simulink model "IPModelNonlinearSystemHomoclinicOrbit"  (R2024a)
settings: Solver=FixedStepAuto  StartTime=0.0  StopTime=80  FixedStep=.01  RelTol=1e-3
PreLoadFcn:
  | m  = .164948;
  | M = 1.035052;
  | l = 0.2425;
  | kdx = 1;
  | kv = 1;
  | kE = 1;
  | kx = 1/100;
  | g = 9.804;
  | 
  | % kdx = kdx*10;
  | % kv = kv*10;
  | % kE = kE*10;
  | % kx = kx*10;
  | %
  | % kdx = kdx*1000;
  | % kv = kv*1000;
  | % kE = kE*1000;
  | % kx = kx*1000;
  | 
  | x0 = 0;
  | dx0 = 0;
  | theta0 = 23*D2R;
  | dtheta0 = 0;
  | 
  | ml = m*l;
  | ml2 = ml*l;
  | 
  | 
  | phi = 25; %error from upright pos, in degrees
  | R2D = 180/pi;
  | D2R = pi/180;
  | 
  | 
  | A = 1/(M*l)*[0 , 1, 0, 0;
  |           0, 0, -m*l*g, 0;
  |           0, 0, 0, 1;
  |           0, 0, (M+m)*g, 0];
  | B = 1/(M*l)*[0;
  |             l;
  |             0;
  |             -1];
  | 
  | C = [1,0,0,0;
  |     0,0,1,0];
  | 
  | D = [0;0];
values from neighbouring files (symbols this model uses):
  K = lqr(A,B,Q,R)    [IPdynamicsHomoclinicOrbitStabilization.m]    (also in invertedPendulumDynamics.m = [-31.6228, -22.4894, 87.1251, 18.1589])
libraries: vrlib x3, simulink x1
settings Model: NumberOfSteps=2  SnapshotBufferSize=5  SnapshotInterval=5  Creator=rahelmizrahi  LastModifiedBy=rahelmizrahi
settings SolverCC: ZeroCrossAlgorithm=Adaptive
settings DebuggingCC: IgnoredZcDiagnostic=none

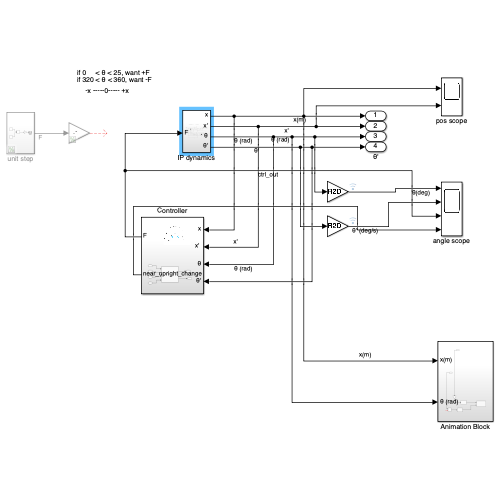
[thumbnail: Simulink's stored preview of the top-level diagram]
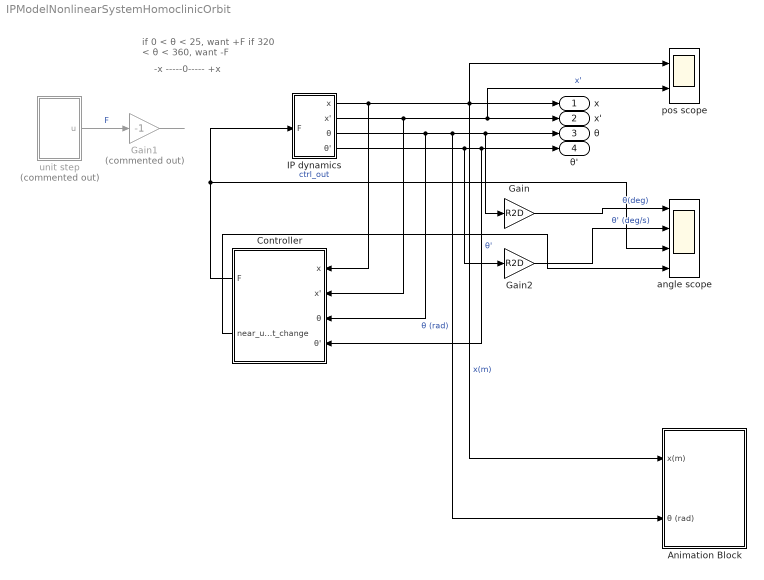
== system IPModelNonlinearSystemHomoclinicOrbit ==
  note: if 0     < θ < 25, want +F
      | if 320 < θ < 360, want -F
  note: -x -----0----- +x
  Animation Block : Subsystem
  Controller : Subsystem
  Gain : Gain  Gain=R2D
  Gain1 : Gain  Commented=on  Gain=-1
  Gain2 : Gain  Gain=R2D
  IP dynamics : Subsystem
  angle scope : Scope  NumInputPorts=4
  pos scope : Scope  NumInputPorts=2
  unit step : Subsystem  Commented=on
  x : Outport
  x' : Outport  Port=2
  θ : Outport  Port=3
  θ' : Outport  Port=4
  wires:
  Gain1/1 -> ?
  IP dynamics/2(x') -> Controller/2("x' "), pos scope/2, x'/1  "x'"
  IP dynamics/4(θ') -> Gain2/1, Controller/4(θ'), θ'/1  "θ'"
  unit step/1(u) -> Gain1/1  "F"
  Gain2/1 -> angle scope/2  "θ' (deg/s)"
  Gain/1 -> angle scope/1  "θ(deg)"
  IP dynamics/3(θ) -> Controller/3(θ), Gain/1, θ/1, Animation Block/2(θ (rad))  "θ (rad)"
  IP dynamics/1(x) -> Animation Block/1(x(m)), pos scope/1, x/1, Controller/1(x)  "x(m)"
  Controller/1(F) -> angle scope/3, IP dynamics/1(F)  "ctrl_out"
  Controller/2(near_upright_change) -> angle scope/4

== system IPModelNonlinearSystemHomoclinicOrbit/Animation Block ==
  x(m) : Inport
  θ (rad) : Inport  Port=2
  Add : Sum
  Gain6 : Gain  Gain=10
  VR Sink1 : vrlib/VR Sink  InstantiateOnLoad=on  SampleTime=0.1  ViewEnable=on  RemoteChange=off  RemoteView=off  FieldsWritten=cart.translation.3.1.1.double#joint.rotation.4.1.1.double  WorldFileName=/Users/rahelmizrahi/Downloads/upload 2/Inverted_pendulum12.wrl  AutoView=on  VideoDimensions=[]  AllowVariableSize=off  FigureProperties="{'Position', 'Name', 'Viewpoint', 'CameraBound', 'CameraDirection', 'CameraPosition', 'CameraUpVector', 'ZoomFactor', 'Antialiasing', 'Headlight', 'Lighting', 'Sound', 'StatusBar', 'Stereo3D', 'Stereo3DCameraOffset', 'Stereo3DHIT', 'ToolBar', 'Textures', 'Transparency', 'Triad', 'Wireframe', 'NavZones', 'NavMode', 'NavSpeed', 'CaptureFileFormat', 'CaptureFileName', 'Record2DCompressMethod', 'Record2DCompressQuality', 'Record2D', 'Record2DFileName', 'Record2DFPS', 'NavPanel'; [5.0000000000000000e+00   1.0300000000000000e+02   5.7600000000000000e+02   3.5000000000000000e+02], '', '', 'on', [0.0000000000000000e+00   0.0000000000000000e+00  -9.9999999999999989e-01], [0.0000000000000000e+00  -6.0000002384185791e-01   2.6254408740997309e+01], [0.0000000000000000e+00   1.0000000000000000e+00   0.0000000000000000e+00], [1.0000000000000000e+00], 'on', 'on', 'on', 'on', 'on', 'off', [1.0000000149011612e-01], [0.0000000000000000e+00], 'on', 'on', 'on', 'none', 'off', 'off', 'fly', 'normal', 'tif', '%f_anim_%n.tif', 'auto', [7.5000000000000000e+01], 'off', '%f_anim_%n.avi', 'auto', 'halfbar'}"
  angle sig expander : vrlib/VR Signal Expander  outwidth=4  outidx=4
  pos sig expander : vrlib/VR Signal Expander  outwidth=3  outidx=1
  wires:
  θ (rad)/1 -> Add/1
  pos sig expander/1 -> VR Sink1/1
  Add/1 -> angle sig expander/1
  ? -> Add/2
  Gain6/1 -> pos sig expander/1
  angle sig expander/1 -> VR Sink1/2
  x(m)/1 -> Gain6/1

== system IPModelNonlinearSystemHomoclinicOrbit/Controller ==
  x : Inport
  "x' " : Inport  Port=2
  θ : Inport  Port=3
  θ' : Inport  Port=4
  ctrl switch : Subsystem
  F : Outport
  near_upright_change : Outport  Port=2
  wires:
  ctrl switch/1(control_out) -> F/1  "F"
  "x' "/1 -> ctrl switch/4("x' ")  "x'"
  x/1 -> ctrl switch/3(x)  "x"
  θ'/1 -> ctrl switch/2(θ')  "θ'"
  θ/1 -> ctrl switch/1(θ)  "θ"
  ctrl switch/2(near_upright_change) -> near_upright_change/1

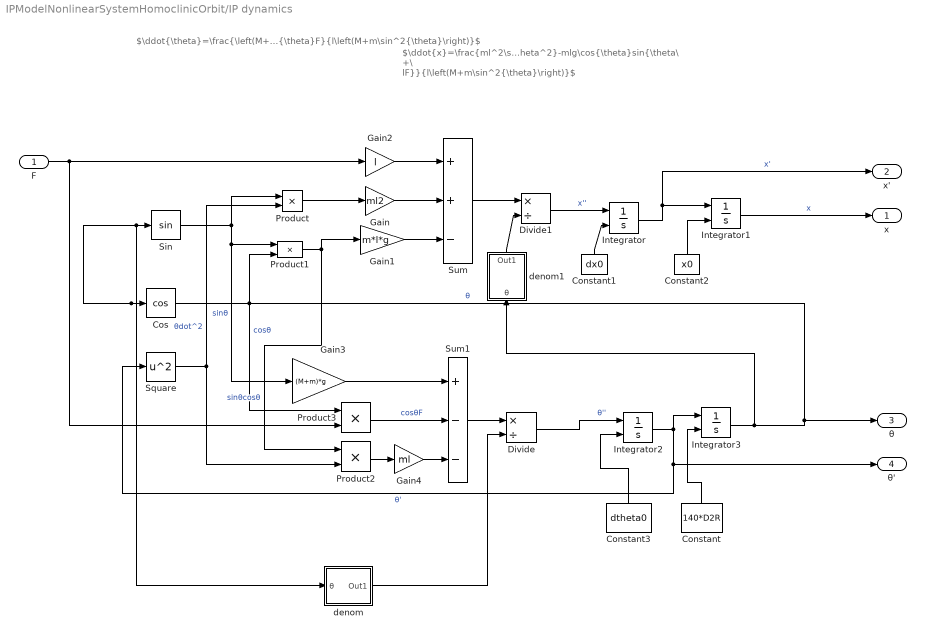
== system IPModelNonlinearSystemHomoclinicOrbit/IP dynamics ==
  note: $\ddot{\theta}=\frac{\left(M+m\right)g\sin{\theta-ml\sin{\theta}\cos{\theta}\dot{\theta^2}}-\cos{\theta}F}{l\left(M+m\sin^2{\theta}\right)}$
  note: $\ddot{x}=\frac{ml^2\sin{\theta}\dot{\theta^2}-mlg\cos{\theta}sin{\theta\ +\ lF}}{l\left(M+m\sin^2{\theta}\right)}$
  F : Inport
  Constant : Constant  Value=140*D2R
  Constant1 : Constant  Value=dx0
  Constant2 : Constant  Value=x0
  Constant3 : Constant  Value=dtheta0
  Cos : Trigonometry  Operator=cos
  Divide : Product  Inputs=*/
  Divide1 : Product  Inputs=*/
  Gain : Gain  Gain=ml2
  Gain1 : Gain  Gain=m*l*g
  Gain2 : Gain  Gain=l
  Gain3 : Gain  Gain=(M+m)*g
  Gain4 : Gain  Gain=ml
  Integrator : Integrator  InitialConditionSource=external
  Integrator1 : Integrator  InitialConditionSource=external
  Integrator2 : Integrator  InitialConditionSource=external
  Integrator3 : Integrator  InitialConditionSource=external  WrappedStateUpperValue=2*pi  WrappedStateLowerValue=0
  Product{,1..3} (4 alike) : Product
  Sin : Trigonometry
  Square : Math  Operator=square
  Sum : Sum  Inputs=++-
  Sum1 : Sum  Inputs=+--
  denom : Subsystem
  denom1 : Subsystem
  x : Outport
  x' : Outport  Port=2
  θ : Outport  Port=3
  θ' : Outport  Port=4
  wires:
  Product/1 -> Gain/1
  Sum1/1 -> Divide/1
  F/1 -> Product3/2, Gain2/1
  Gain2/1 -> Sum/1
  Product1/1 -> Product2/1, Gain1/1  "sinθcosθ"
  Product3/1 -> Sum1/2  "cosθF"
  Gain1/1 -> Sum/3
  Integrator1/1 -> x/1  "x"
  Square/1 -> Product/2, Product2/2  "θdot^2"
  Cos/1 -> Product1/2, Product3/1  "cosθ"
  Integrator2/1 -> Integrator3/1, θ'/1, Square/1  "θ'"
  Integrator3/1 -> denom1/1(θ), θ/1, denom/1(θ), Sin/1, Cos/1  "θ"
  Gain3/1 -> Sum1/1
  Gain/1 -> Sum/2
  Product2/1 -> Gain4/1
  Sin/1 -> Gain3/1, Product1/1, Product/1  "sinθ"
  Integrator/1 -> x'/1, Integrator1/1  "x'"
  Sum/1 -> Divide1/1
  Gain4/1 -> Sum1/3
  Constant/1 -> Integrator3/2
  Constant1/1 -> Integrator/2
  Constant2/1 -> Integrator1/2
  Constant3/1 -> Integrator2/2
  Divide/1 -> Integrator2/1  "θ''"
  denom/1(Out1) -> Divide/2
  Divide1/1 -> Integrator/1  "x''"
  denom1/1(Out1) -> Divide1/2

== system IPModelNonlinearSystemHomoclinicOrbit/unit step ==
  Add : Sum  Inputs=-+
  Gain : Gain  Gain=10
  Step : Step  SampleTime=0
  Step1 : Step  Time=1.1  SampleTime=0
  u : Outport
  wires:
  Step1/1 -> Add/1
  Gain/1 -> u/1
  Step/1 -> Add/2
  Add/1 -> Gain/1

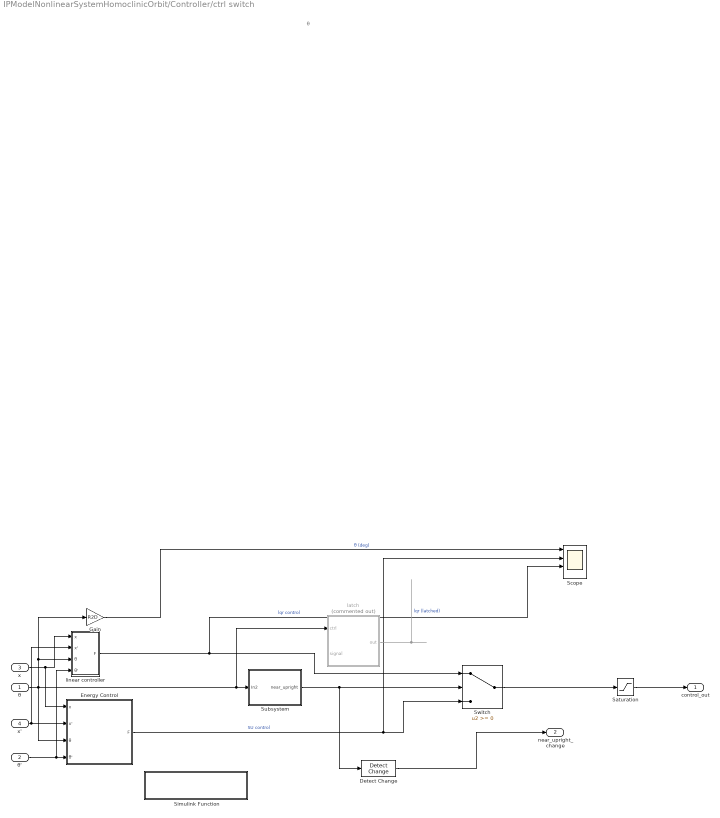
== system IPModelNonlinearSystemHomoclinicOrbit/Controller/ctrl switch ==
  note: θ
  θ : Inport
  θ' : Inport  Port=2
  x : Inport  Port=3
  "x' " : Inport  Port=4
  Detect Change : simulink/Logic and Bit Operations/Detect Change  vinit=0  OutDataTypeStr=boolean
  Energy Control : Subsystem
  Gain : Gain  Gain=R2D
  Saturation : Saturate  UpperLimit=6  LowerLimit=-6
  Scope : Scope  NumInputPorts=4
  Simulink Function : Subsystem  TreatAsAtomicUnit=on
  Subsystem : Subsystem
  Switch : Switch  SaturateOnIntegerOverflow=off  InputSameDT=off
  latch : Subsystem  Commented=on
  linear controller : Subsystem
  control_out : Outport
  near_upright_change : Outport  Port=2
  wires:
  Subsystem/1(near_upright) -> Detect Change/1, Switch/2
  Energy Control/1(F) -> Scope/2, Switch/3  "SU control"
  θ'/1 -> linear controller/4(θ'), Energy Control/4(θ')
  linear controller/1(F) -> Scope/3, Switch/1  "lqr control"
  "x' "/1 -> linear controller/2(x'), Energy Control/2(x')
  x/1 -> linear controller/1(x), Energy Control/1(x)
  θ/1 -> linear controller/3(θ), Gain/1, Energy Control/3(θ), latch/1(ctrl), Subsystem/1(In2)
  latch/1(out) -> ?  "lqr (latched)"
  Gain/1 -> Scope/1  "θ (deg)"
  Detect Change/1 -> near_upright_change/1
  Switch/1 -> Saturation/1
  Saturation/1 -> control_out/1

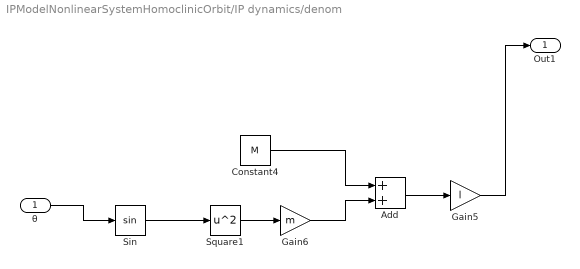
== system IPModelNonlinearSystemHomoclinicOrbit/IP dynamics/denom ==
  θ : Inport
  Add : Sum
  Constant4 : Constant  Value=M
  Gain5 : Gain  Gain=l
  Gain6 : Gain  Gain=m
  Sin : Trigonometry
  Square1 : Math  Operator=square
  Out1 : Outport
  wires:
  Gain5/1 -> Out1/1
  Square1/1 -> Gain6/1
  θ/1 -> Sin/1
  Constant4/1 -> Add/1
  Add/1 -> Gain5/1
  Gain6/1 -> Add/2
  Sin/1 -> Square1/1

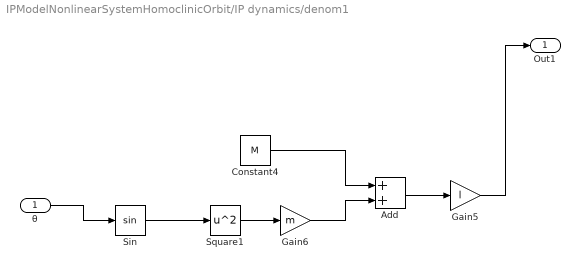
== system IPModelNonlinearSystemHomoclinicOrbit/IP dynamics/denom1 ==
  θ : Inport
  Add : Sum
  Constant4 : Constant  Value=M
  Gain5 : Gain  Gain=l
  Gain6 : Gain  Gain=m
  Sin : Trigonometry
  Square1 : Math  Operator=square
  Out1 : Outport
  wires:
  Gain5/1 -> Out1/1
  Square1/1 -> Gain6/1
  θ/1 -> Sin/1
  Constant4/1 -> Add/1
  Add/1 -> Gain5/1
  Gain6/1 -> Add/2
  Sin/1 -> Square1/1

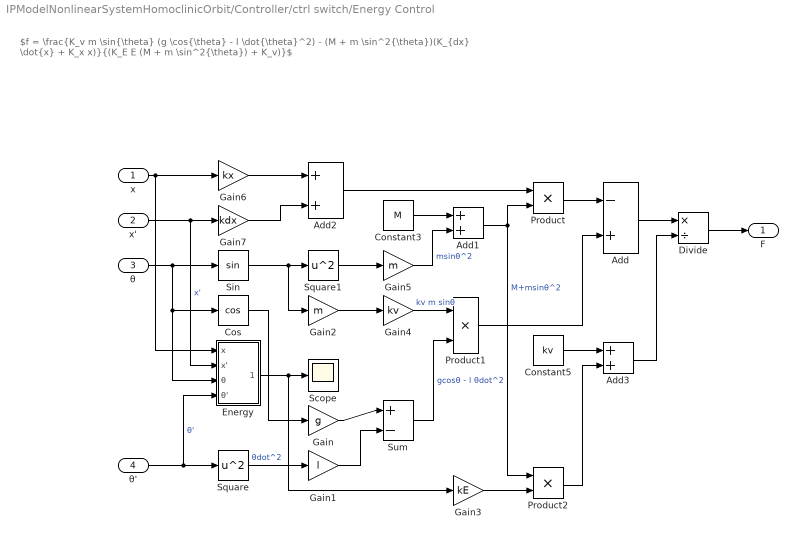
== system IPModelNonlinearSystemHomoclinicOrbit/Controller/ctrl switch/Energy Control ==
  note: $f = \frac{K_v m \sin{\theta} (g \cos{\theta} - l \dot{\theta}^2) - (M + m \sin^2{\theta})(K_{dx} \dot{x} + K_x x)}{(K_E E (M + m \sin^2{\theta}) + K_v)}$
  x : Inport
  x' : Inport  Port=2
  θ : Inport  Port=3
  θ' : Inport  Port=4
  Add : Sum  Inputs=-+
  Add1 : Sum
  Add2 : Sum
  Add3 : Sum
  Constant3 : Constant  Value=M
  Constant5 : Constant  Value=kv
  Cos : Trigonometry  Operator=cos
  Divide : Product  Inputs=*/
  Energy : Subsystem
  Gain : Gain  Gain=g
  Gain1 : Gain  Gain=l
  Gain2 : Gain  Gain=m
  Gain3 : Gain  Gain=kE
  Gain4 : Gain  Gain=kv
  Gain5 : Gain  Gain=m
  Gain6 : Gain  Gain=kx
  Gain7 : Gain  Gain=kdx
  Product : Product
  Product1 : Product
  Product2 : Product
  Scope : Scope
  Sin : Trigonometry
  Square : Math  Operator=square
  Square1 : Math  Operator=square
  Sum : Sum  Inputs=|+-
  F : Outport
  wires:
  Add/1 -> Divide/1
  Gain3/1 -> Product2/2
  Square/1 -> Gain1/1  "θdot^2"
  Add1/1 -> Product/2, Product2/1  "M+msinθ^2"
  Product/1 -> Add/1
  Sum/1 -> Product1/2  "gcosθ - l θdot^2"
  Gain4/1 -> Product1/1  "kv m sinθ"
  θ/1 -> Energy/3(θ), Cos/1, Sin/1
  Constant3/1 -> Add1/1
  Gain1/1 -> Sum/2
  Gain/1 -> Sum/1
  Add3/1 -> Divide/2
  x'/1 -> Energy/2(x'), Gain7/1  "x'"
  Product1/1 -> Add/2
  Gain2/1 -> Gain4/1
  Cos/1 -> Gain/1
  Add2/1 -> Product/1
  Gain6/1 -> Add2/1
  Square1/1 -> Gain5/1
  Energy/1(Energy) -> Scope/1, Gain3/1
  Gain7/1 -> Add2/2
  Product2/1 -> Add3/2
  Constant5/1 -> Add3/1
  θ'/1 -> Square/1, Energy/4(θ')  "θ'"
  Gain5/1 -> Add1/2  "msinθ^2"
  Divide/1 -> F/1
  x/1 -> Energy/1(x), Gain6/1
  Sin/1 -> Gain2/1, Square1/1

== system IPModelNonlinearSystemHomoclinicOrbit/Controller/ctrl switch/Simulink Function ==
  between : TriggerPort  TriggerType=function-call  IsSimulinkFunction=on  FunctionName=between  FunctionVisibility=scoped  VariantControl=(inherit)
  AND : Logic  IconShape=distinctive  AllPortsSameDT=off  OutDataTypeStr=boolean
  Relational Operator : RelationalOperator  OutDataTypeStr=boolean  RndMeth=Simplest  InputSameDT=off
  Relational Operator1 : RelationalOperator  Operator=<=  OutDataTypeStr=boolean  RndMeth=Simplest  InputSameDT=off
  input : ArgIn  DisableCoverage=on  ArgumentName=input
  min : ArgIn  Port=2  ArgumentName=min
  max : ArgIn  Port=3  ArgumentName=max
  out : ArgOut  DisableCoverage=on  OutDataTypeStr=boolean  ArgumentName=out
  wires:
  input/1 -> Relational Operator1/1, Relational Operator/1
  Relational Operator/1 -> AND/1
  Relational Operator1/1 -> AND/2
  AND/1 -> out/1
  min/1 -> Relational Operator/2
  max/1 -> Relational Operator1/2

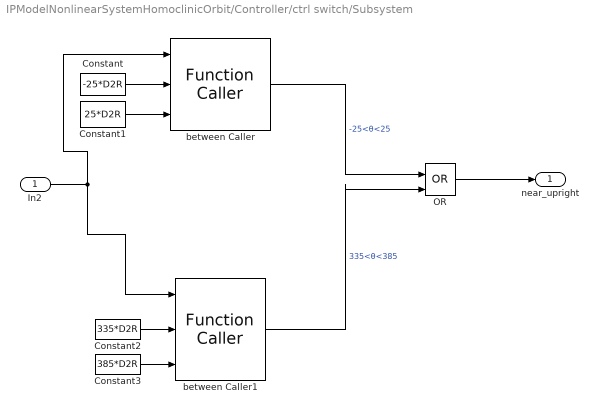
== system IPModelNonlinearSystemHomoclinicOrbit/Controller/ctrl switch/Subsystem ==
  In2 : Inport
  Constant : Constant  Value=-25*D2R
  Constant1 : Constant  Value=25*D2R
  Constant2 : Constant  Value=335*D2R
  Constant3 : Constant  Value=385*D2R
  OR : Logic  Operator=OR  IconShape=distinctive  AllPortsSameDT=off  OutDataTypeStr=boolean
  between Caller : FunctionCaller  FunctionPrototype=out = between(input,min,max)  InputArgumentSpecifications=double(1), double(1), double(1)  OutputArgumentSpecifications=boolean(1)
  between Caller1 : FunctionCaller  FunctionPrototype=out = between(input,min,max)  InputArgumentSpecifications=double(1), double(1), double(1)  OutputArgumentSpecifications=boolean(1)
  near_upright : Outport
  wires:
  In2/1 -> between Caller1/1, between Caller/1
  between Caller1/1 -> OR/2  "335<θ<385"
  Constant3/1 -> between Caller1/3
  Constant1/1 -> between Caller/3
  between Caller/1 -> OR/1  "-25<θ<25"
  Constant/1 -> between Caller/2
  Constant2/1 -> between Caller1/2
  OR/1 -> near_upright/1

== system IPModelNonlinearSystemHomoclinicOrbit/Controller/ctrl switch/latch ==
  ctrl : Inport
  signal : Inport  Port=2
  Memory : Memory
  Switch1 : Switch  Criteria=u2 ~= 0  SaturateOnIntegerOverflow=off  InputSameDT=off
  out : Outport
  wires:
  signal/1 -> Switch1/1
  Memory/1 -> Switch1/3
  Switch1/1 -> out/1, Memory/1
  ctrl/1 -> Switch1/2

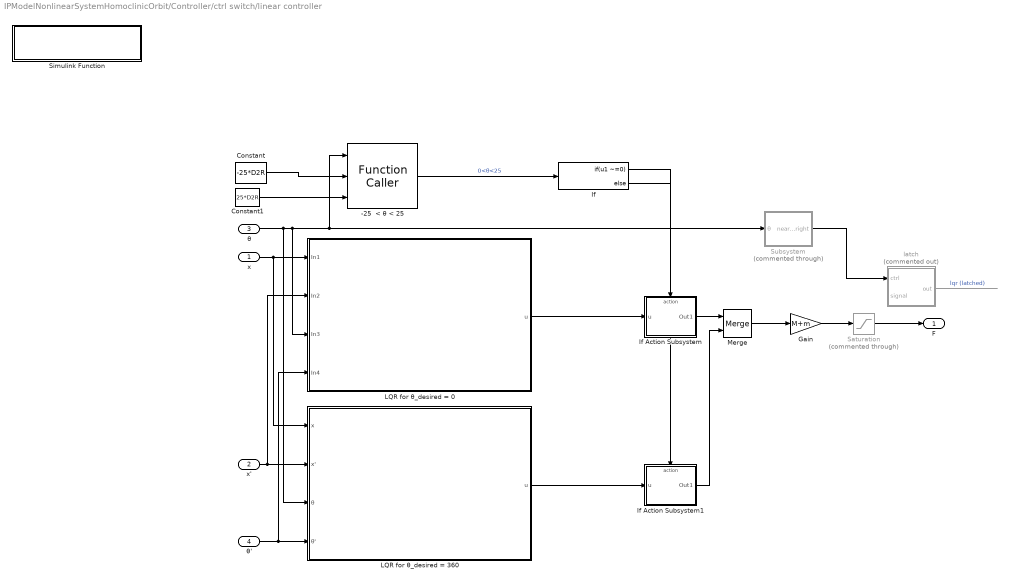
== system IPModelNonlinearSystemHomoclinicOrbit/Controller/ctrl switch/linear controller ==
  x : Inport
  x' : Inport  Port=2
  θ : Inport  Port=3
  θ' : Inport  Port=4
  -25  < θ < 25 : FunctionCaller  FunctionPrototype=out = between(input,min,max)  InputArgumentSpecifications=double(1), double(1), double(1)  OutputArgumentSpecifications=boolean(1)
  Constant : Constant  Value=-25*D2R
  Constant1 : Constant  Value=25*D2R
  Gain : Gain  Gain=M+m
  If : If  IfExpression=u1 ~=0
  If Action Subsystem : Subsystem  TreatAsAtomicUnit=on
  If Action Subsystem1 : Subsystem  TreatAsAtomicUnit=on
  LQR for θ_desired = 0 : Subsystem
  LQR for θ_desired = 360 : Subsystem
  Merge : Merge
  Saturation : Saturate  Commented=through  UpperLimit=5  LowerLimit=-5
  Simulink Function : Subsystem  TreatAsAtomicUnit=on
  Subsystem : Subsystem  Commented=through
  latch : Subsystem  Commented=on
  F : Outport
  wires:
  Merge/1 -> Gain/1
  If Action Subsystem/1(Out1) -> Merge/1
  x/1 -> LQR for θ_desired = 0/1(In1), LQR for θ_desired = 360/1(x)
  x'/1 -> LQR for θ_desired = 0/2(In2), LQR for θ_desired = 360/2(x')
  LQR for θ_desired = 360/1(u) -> If Action Subsystem1/1(u)
  -25  < θ < 25/1 -> If/1  "0<θ<25"
  θ'/1 -> LQR for θ_desired = 0/4(In4), LQR for θ_desired = 360/4(θ')
  If/1 -> If Action Subsystem/Action
  If/2 -> If Action Subsystem1/Action
  θ/1 -> Subsystem/1(θ), -25  < θ < 25/1, LQR for θ_desired = 0/3(In3), LQR for θ_desired = 360/3(θ)
  If Action Subsystem1/1(Out1) -> Merge/2
  Constant1/1 -> -25  < θ < 25/3
  Constant/1 -> -25  < θ < 25/2
  Subsystem/1(near_upright) -> latch/1(ctrl)
  latch/1(out) -> ?  "lqr (latched)"
  Saturation/1 -> F/1
  Gain/1 -> Saturation/1
  LQR for θ_desired = 0/1(u) -> If Action Subsystem/1(u)

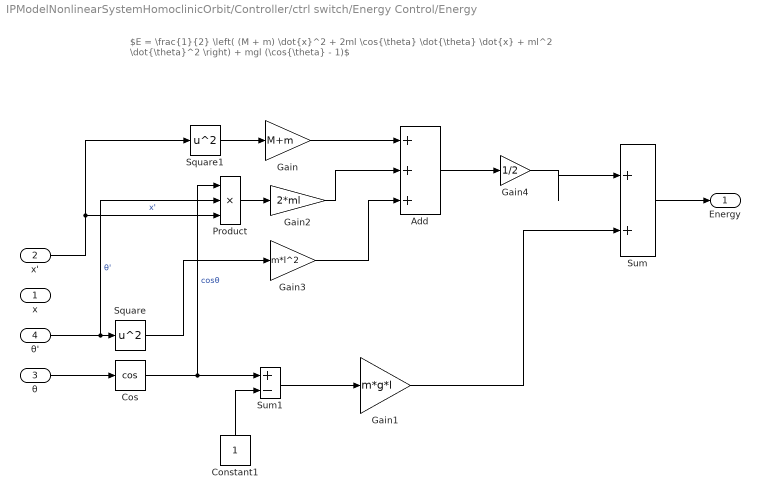
== system IPModelNonlinearSystemHomoclinicOrbit/Controller/ctrl switch/Energy Control/Energy ==
  note: $E = \frac{1}{2} \left( (M + m) \dot{x}^2 + 2ml \cos{\theta} \dot{\theta} \dot{x} + ml^2 \dot{\theta}^2 \right) + mgl (\cos{\theta} - 1)$
  x : Inport
  x' : Inport  Port=2
  θ : Inport  Port=3
  θ' : Inport  Port=4
  Add : Sum  Inputs=+++
  Constant1 : Constant
  Cos : Trigonometry  Operator=cos
  Gain : Gain  Gain=M+m
  Gain1 : Gain  Gain=m*g*l
  Gain2 : Gain  Gain=2*ml
  Gain3 : Gain  Gain=m*l^2
  Gain4 : Gain  Gain=1/2
  Product : Product  Inputs=3
  Square : Math  Operator=square
  Square1 : Math  Operator=square
  Sum : Sum  Inputs=|++
  Sum1 : Sum  Inputs=+-
  Energy : Outport
  wires:
  θ/1 -> Cos/1
  Constant1/1 -> Sum1/2
  Square/1 -> Gain3/1
  Sum1/1 -> Gain1/1
  θ'/1 -> Product/2, Square/1  "θ'"
  Cos/1 -> Product/1, Sum1/1  "cosθ"
  Gain1/1 -> Sum/2
  Square1/1 -> Gain/1
  x'/1 -> Product/3, Square1/1  "x'"
  Gain/1 -> Add/1
  Product/1 -> Gain2/1
  Gain2/1 -> Add/2
  Gain3/1 -> Add/3
  Add/1 -> Gain4/1
  Gain4/1 -> Sum/1
  Sum/1 -> Energy/1

== system IPModelNonlinearSystemHomoclinicOrbit/Controller/ctrl switch/linear controller/If Action Subsystem ==
  u : Inport
  Action Port : ActionPort  ActionPortLabel=if(u1 ~=0)
  Out1 : Outport
  wires:
  u/1 -> Out1/1

== system IPModelNonlinearSystemHomoclinicOrbit/Controller/ctrl switch/linear controller/If Action Subsystem1 ==
  u : Inport
  Action Port : ActionPort  ActionPortLabel=else
  Out1 : Outport
  wires:
  u/1 -> Out1/1

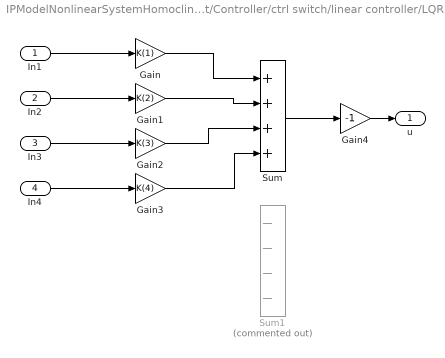
== system IPModelNonlinearSystemHomoclinicOrbit/Controller/ctrl switch/linear controller/LQR for θ_desired = 0 ==
  In1 : Inport
  In2 : Inport  Port=2
  In3 : Inport  Port=3
  In4 : Inport  Port=4
  Gain : Gain  Gain=K(1)
  Gain1 : Gain  Gain=K(2)
  Gain2 : Gain  Gain=K(3)
  Gain3 : Gain  Gain=K(4)
  Gain4 : Gain  Gain=-1
  Sum : Sum  Inputs=++++
  Sum1 : Sum  Commented=on  Inputs=----
  u : Outport
  wires:
  In4/1 -> Gain3/1
  In2/1 -> Gain1/1
  Gain1/1 -> Sum/2
  Gain3/1 -> Sum/4
  Sum/1 -> Gain4/1
  Gain2/1 -> Sum/3
  In3/1 -> Gain2/1
  In1/1 -> Gain/1
  Gain/1 -> Sum/1
  Gain4/1 -> u/1

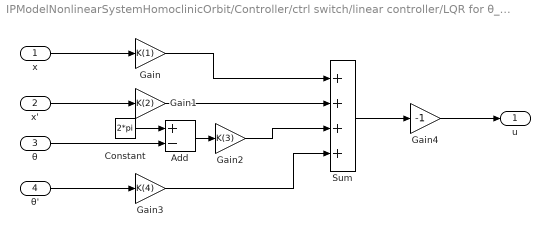
== system IPModelNonlinearSystemHomoclinicOrbit/Controller/ctrl switch/linear controller/LQR for θ_desired = 360 ==
  x : Inport
  x' : Inport  Port=2
  θ : Inport  Port=3
  θ' : Inport  Port=4
  Add : Sum  Inputs=+-
  Constant : Constant  Value=2*pi
  Gain : Gain  Gain=K(1)
  Gain1 : Gain  Gain=K(2)
  Gain2 : Gain  Gain=K(3)
  Gain3 : Gain  Gain=K(4)
  Gain4 : Gain  Gain=-1
  Sum : Sum  Inputs=++++
  u : Outport
  wires:
  θ'/1 -> Gain3/1
  x'/1 -> Gain1/1
  Gain1/1 -> Sum/2
  Gain3/1 -> Sum/4
  Sum/1 -> Gain4/1
  θ/1 -> Add/2
  x/1 -> Gain/1
  Gain/1 -> Sum/1
  Constant/1 -> Add/1
  Add/1 -> Gain2/1
  Gain2/1 -> Sum/3
  Gain4/1 -> u/1

== system IPModelNonlinearSystemHomoclinicOrbit/Controller/ctrl switch/linear controller/Simulink Function ==
  between : TriggerPort  TriggerType=function-call  IsSimulinkFunction=on  FunctionName=between  FunctionVisibility=scoped  VariantControl=(inherit)
  AND : Logic  IconShape=distinctive  AllPortsSameDT=off  OutDataTypeStr=boolean
  Relational Operator : RelationalOperator  OutDataTypeStr=boolean  RndMeth=Simplest  InputSameDT=off
  Relational Operator1 : RelationalOperator  Operator=<=  OutDataTypeStr=boolean  RndMeth=Simplest  InputSameDT=off
  input : ArgIn  DisableCoverage=on  ArgumentName=input
  min : ArgIn  Port=2  ArgumentName=min
  max : ArgIn  Port=3  ArgumentName=max
  out : ArgOut  DisableCoverage=on  OutDataTypeStr=boolean  ArgumentName=out
  wires:
  input/1 -> Relational Operator1/1, Relational Operator/1
  Relational Operator/1 -> AND/1
  Relational Operator1/1 -> AND/2
  AND/1 -> out/1
  min/1 -> Relational Operator/2
  max/1 -> Relational Operator1/2

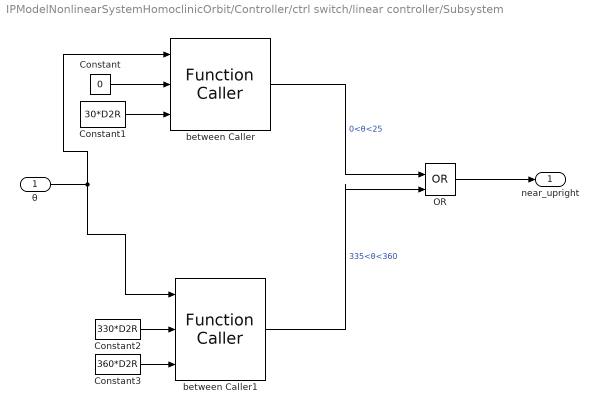
== system IPModelNonlinearSystemHomoclinicOrbit/Controller/ctrl switch/linear controller/Subsystem ==
  θ : Inport
  Constant : Constant  Value=0
  Constant1 : Constant  Value=30*D2R
  Constant2 : Constant  Value=330*D2R
  Constant3 : Constant  Value=360*D2R
  OR : Logic  Operator=OR  IconShape=distinctive  AllPortsSameDT=off  OutDataTypeStr=boolean
  between Caller : FunctionCaller  FunctionPrototype=out = between(input,min,max)  InputArgumentSpecifications=double(1), double(1), double(1)  OutputArgumentSpecifications=boolean(1)
  between Caller1 : FunctionCaller  FunctionPrototype=out = between(input,min,max)  InputArgumentSpecifications=double(1), double(1), double(1)  OutputArgumentSpecifications=boolean(1)
  near_upright : Outport
  wires:
  θ/1 -> between Caller1/1, between Caller/1
  between Caller1/1 -> OR/2  "335<θ<360"
  Constant3/1 -> between Caller1/3
  Constant1/1 -> between Caller/3
  between Caller/1 -> OR/1  "0<θ<25"
  Constant/1 -> between Caller/2
  Constant2/1 -> between Caller1/2
  OR/1 -> near_upright/1

== system IPModelNonlinearSystemHomoclinicOrbit/Controller/ctrl switch/linear controller/latch ==
  ctrl : Inport
  signal : Inport  Port=2
  Memory : Memory
  Switch1 : Switch  Criteria=u2 ~= 0  SaturateOnIntegerOverflow=off  InputSameDT=off
  out : Outport
  wires:
  signal/1 -> Switch1/1
  Memory/1 -> Switch1/3
  Switch1/1 -> out/1, Memory/1
  ctrl/1 -> Switch1/2
